simulink model "PI_controller"  (R2020b)
settings: Solver=VariableStepAuto  StartTime=0.0  StopTime=10.0  RelTol=1e-3
model workspace (MAT data in the model file):
  ki = Simulink.Parameter
  ki.Value = 10
  ki.DataType = 'auto'
  ki.Dimensions = [1 1]
  kp = Simulink.Parameter
  kp.Value = 10
  kp.DataType = 'auto'
  kp.Dimensions = [1 1]
  ts = Simulink.Parameter
  ts.Value = 1
  ts.DataType = 'auto'
  ts.Dimensions = [1 1]
settings Model: Creator=SAGAR  LastModifiedBy=SAGAR
settings DataIOCC: SaveOutput=off  SaveTime=off

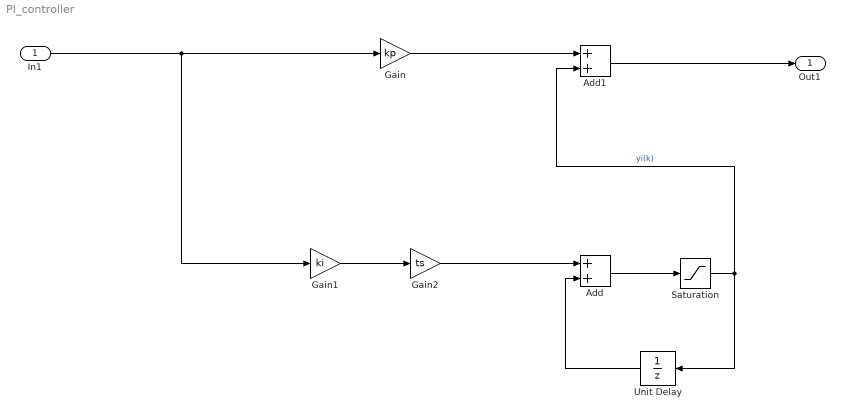
== system PI_controller ==
  In1 : Inport  OutDataTypeStr=double  PortDimensions=1  SampleTime=[0,1]
  Add : Sum
  Add1 : Sum
  Gain : Gain  Gain=kp
  Gain1 : Gain  Gain=ki
  Gain2 : Gain  Gain=ts
  Saturation : Saturate  UpperLimit=1  LowerLimit=-1
  Unit Delay : UnitDelay  SampleTime=-1  HasFrameUpgradeWarning=on
  Out1 : Outport  OutDataTypeStr=double  PortDimensions=1  SampleTime=[0,1]
  wires:
  Gain1/1 -> Gain2/1
  Add/1 -> Saturation/1
  Add1/1 -> Out1/1
  Unit Delay/1 -> Add/2
  Saturation/1 -> Unit Delay/1, Add1/2  "yi(k)"
  In1/1 -> Gain/1, Gain1/1
  Gain/1 -> Add1/1
  Gain2/1 -> Add/1
